simulink model "demo"  (R2021b)
settings: Solver=VariableStepAuto  StartTime=0.0  StopTime=10  RelTol=1e-3
undefined symbols (not defined in the file or in its folder): xc7vx485tffg1157
libraries: hdlBasic x1736, vmcUtilities x1
(part 6 of 7)

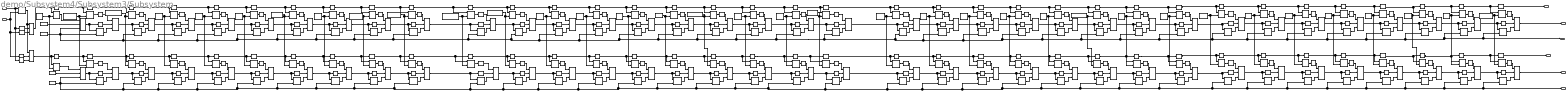
== system demo/Subsystem4/Subsystem3/Subsystem ==
  note: 30
  note: 20
  note: tmp_3
  note: ooki
  note: 10
  note: tmp_2
  note: tiisai
  note: 01
  In1 : Inport
  In2 : Inport  Port=2
  AddSub{,1..17,23..38,41..61,70..79,87,97,108,110..111} (70 alike) : hdlBasic/AddSub  mode=Addition  use_carryin=off  use_carryout=off  en=off  latency=1  precision=User Defined  arith_type="Signed  (2's comp)"  n_bits=32  bin_pt=0  quantization=Truncate  overflow=Wrap  use_behavioral_HDL=off  hw_selection=Fabric  pipelined=off  XmcBlockStatus=1  maskContainerNames=tabcontainer1  block_type=addsub  block_config=sysgen:Addsub_config
  Constant1 : hdlBasic/Constant  const=0  gui_display_data_type=Fixed-point  arith_type=Signed (2's comp)  n_bits=32  bin_pt=0  preci_type=Single  exp_width=8  frac_width=24  explicit_period=on  period=1  XmcBlockStatus=1  maskContainerNames=tabcontainer1  block_type=constant  block_config=sysgen:Constant_config
  Constant2 : hdlBasic/Constant  const=1  gui_display_data_type=Fixed-point  arith_type=Signed (2's comp)  n_bits=32  bin_pt=0  preci_type=Single  exp_width=8  frac_width=24  explicit_period=on  period=1  XmcBlockStatus=1  maskContainerNames=tabcontainer1  block_type=constant  block_config=sysgen:Constant_config
  Constant6 : hdlBasic/Constant  const=0  gui_display_data_type=Fixed-point  arith_type=Signed (2's comp)  n_bits=32  bin_pt=0  preci_type=Single  exp_width=8  frac_width=24  explicit_period=on  period=1  XmcBlockStatus=1  maskContainerNames=tabcontainer1  block_type=constant  block_config=sysgen:Constant_config
  Constant7 : hdlBasic/Constant  const=1  gui_display_data_type=Fixed-point  arith_type=Signed (2's comp)  n_bits=32  bin_pt=0  preci_type=Single  exp_width=8  frac_width=24  explicit_period=on  period=1  XmcBlockStatus=1  maskContainerNames=tabcontainer1  block_type=constant  block_config=sysgen:Constant_config
  Delay{1..7,9..10,12..13,15..16,19..20,22..23,25..26,28..29,31..32,34..35,37..38,41..42,44..45,47..48,50..52,54..56,58,62,64..65,67..68,71..72,74..75,77..78,80..82,84..85,87..88,91..92,94..95,97..98,100..103,105..107,109,114..115,117..118,120..125,127..129,131,133..134,136..138,140..141,143..144,147..148,150..151,153..154,156..158,160..161,163..164,167..168,170..171,173..174,176,188..189,194,205,227,238,257..258,260..261,263..264,266..267,269..270,272..273,275..276,279..280,282..283,285..286,288..290,292,321} (146 alike) : hdlBasic/Delay  rst=off  en=off  latency=1  reg_retiming=off  XmcBlockStatus=1  maskContainerNames=group1  block_type=delay  block_config=sysgen:Delay_config
  Delay{8,11,14,17..18,21,24,27,30,33,36,39..40,43,46,49,53,57,63,66,69..70,73,76,79,83,86,89..90,93,96,99,104,108,116,119,126,130,132,135,139,142,145..146,149,152,155,159,162,165..166,169,172,175,187,216,249,256,259,262,265,268,271,274,277..278,281,284,287,291} (70 alike) : hdlBasic/Delay  rst=off  en=off  latency=2  reg_retiming=off  XmcBlockStatus=1  maskContainerNames=group1  block_type=delay  block_config=sysgen:Delay_config
  Mux{,1..37,40..57,68..77,86,97,106..109} (72 alike) : hdlBasic/Mux  inputs=2  en=off  latency=1  precision=Full  arith_type=Unsigned  n_bits=16  bin_pt=14  quantization=Truncate  overflow=Wrap  XmcBlockStatus=1  maskContainerNames=tabcontainer1  block_type=mux  block_config=sysgen:Mux_config
  Relational : hdlBasic/Relational  mode=a<b  op_type=Bool  en=off  latency=1  XmcBlockStatus=1  maskContainerNames=tabcontainer1  block_type=relational  block_config=sysgen:Relational_config
  Relational{1..36,39..59,70..78,86,97,107..110} (72 alike) : hdlBasic/Relational  mode=a>=b  op_type=Bool  en=off  latency=1  XmcBlockStatus=1  maskContainerNames=tabcontainer1  block_type=relational  block_config=sysgen:Relational_config
  logi_b0 : hdlBasic/Constant  const=-1.0000000000000000000000000000000000000000000000000000000  gui_display_data_type=Floating-point  arith_type=Floating-point  n_bits=8  bin_pt=8  preci_type=Double  exp_width=8  frac_width=24  explicit_period=on  period=1  XmcBlockStatus=1  maskContainerNames=tabcontainer1  block_type=constant  block_config=sysgen:Constant_config
  logi_b1 : hdlBasic/Constant  const=-0.9838709677419354981964261241955682635307312011718750000  gui_display_data_type=Floating-point  arith_type=Floating-point  n_bits=8  bin_pt=8  preci_type=Double  exp_width=8  frac_width=24  explicit_period=on  period=1  XmcBlockStatus=1  maskContainerNames=tabcontainer1  block_type=constant  block_config=sysgen:Constant_config
  logi_b10 : hdlBasic/Constant  const=-0.8387096774193547599196563169243745505809783935546875000  gui_display_data_type=Floating-point  arith_type=Floating-point  n_bits=8  bin_pt=8  preci_type=Double  exp_width=8  frac_width=24  explicit_period=on  period=1  XmcBlockStatus=1  maskContainerNames=tabcontainer1  block_type=constant  block_config=sysgen:Constant_config
  logi_b11 : hdlBasic/Constant  const=-0.8225806451612902581160824411199428141117095947265625000  gui_display_data_type=Floating-point  arith_type=Floating-point  n_bits=8  bin_pt=8  preci_type=Double  exp_width=8  frac_width=24  explicit_period=on  period=1  XmcBlockStatus=1  maskContainerNames=tabcontainer1  block_type=constant  block_config=sysgen:Constant_config
  logi_b12 : hdlBasic/Constant  const=-0.8064516129032257563125085653155110776424407958984375000  gui_display_data_type=Floating-point  arith_type=Floating-point  n_bits=8  bin_pt=8  preci_type=Double  exp_width=8  frac_width=24  explicit_period=on  period=1  XmcBlockStatus=1  maskContainerNames=tabcontainer1  block_type=constant  block_config=sysgen:Constant_config
  logi_b13 : hdlBasic/Constant  const=-0.7903225806451612545089346895110793411731719970703125000  gui_display_data_type=Floating-point  arith_type=Floating-point  n_bits=8  bin_pt=8  preci_type=Double  exp_width=8  frac_width=24  explicit_period=on  period=1  XmcBlockStatus=1  maskContainerNames=tabcontainer1  block_type=constant  block_config=sysgen:Constant_config
  logi_b14 : hdlBasic/Constant  const=-0.7741935483870967527053608137066476047039031982421875000  gui_display_data_type=Floating-point  arith_type=Floating-point  n_bits=8  bin_pt=8  preci_type=Double  exp_width=8  frac_width=24  explicit_period=on  period=1  XmcBlockStatus=1  maskContainerNames=tabcontainer1  block_type=constant  block_config=sysgen:Constant_config
  logi_b15 : hdlBasic/Constant  const=-0.7580645161290322509017869379022158682346343994140625000  gui_display_data_type=Floating-point  arith_type=Floating-point  n_bits=8  bin_pt=8  preci_type=Double  exp_width=8  frac_width=24  explicit_period=on  period=1  XmcBlockStatus=1  maskContainerNames=tabcontainer1  block_type=constant  block_config=sysgen:Constant_config
  logi_b16 : hdlBasic/Constant  const=-0.7419354838709677490982130620977841317653656005859375000  gui_display_data_type=Floating-point  arith_type=Floating-point  n_bits=8  bin_pt=8  preci_type=Double  exp_width=8  frac_width=24  explicit_period=on  period=1  XmcBlockStatus=1  maskContainerNames=tabcontainer1  block_type=constant  block_config=sysgen:Constant_config
  logi_b17 : hdlBasic/Constant  const=-0.7258064516129032472946391862933523952960968017578125000  gui_display_data_type=Floating-point  arith_type=Floating-point  n_bits=8  bin_pt=8  preci_type=Double  exp_width=8  frac_width=24  explicit_period=on  period=1  XmcBlockStatus=1  maskContainerNames=tabcontainer1  block_type=constant  block_config=sysgen:Constant_config
  logi_b18 : hdlBasic/Constant  const=-0.7096774193548387454910653104889206588268280029296875000  gui_display_data_type=Floating-point  arith_type=Floating-point  n_bits=8  bin_pt=8  preci_type=Double  exp_width=8  frac_width=24  explicit_period=on  period=1  XmcBlockStatus=1  maskContainerNames=tabcontainer1  block_type=constant  block_config=sysgen:Constant_config
  logi_b19 : hdlBasic/Constant  const=-0.6935483870967741326651889721688348799943923950195312500  gui_display_data_type=Floating-point  arith_type=Floating-point  n_bits=8  bin_pt=8  preci_type=Double  exp_width=8  frac_width=24  explicit_period=on  period=1  XmcBlockStatus=1  maskContainerNames=tabcontainer1  block_type=constant  block_config=sysgen:Constant_config
  logi_b2 : hdlBasic/Constant  const=-0.9677419354838709963928522483911365270614624023437500000  gui_display_data_type=Floating-point  arith_type=Floating-point  n_bits=8  bin_pt=8  preci_type=Double  exp_width=8  frac_width=24  explicit_period=on  period=1  XmcBlockStatus=1  maskContainerNames=tabcontainer1  block_type=constant  block_config=sysgen:Constant_config
  logi_b20 : hdlBasic/Constant  const=-0.6774193548387096308616150963644031435251235961914062500  gui_display_data_type=Floating-point  arith_type=Floating-point  n_bits=8  bin_pt=8  preci_type=Double  exp_width=8  frac_width=24  explicit_period=on  period=1  XmcBlockStatus=1  maskContainerNames=tabcontainer1  block_type=constant  block_config=sysgen:Constant_config
  logi_b21 : hdlBasic/Constant  const=-0.6612903225806451290580412205599714070558547973632812500  gui_display_data_type=Floating-point  arith_type=Floating-point  n_bits=8  bin_pt=8  preci_type=Double  exp_width=8  frac_width=24  explicit_period=on  period=1  XmcBlockStatus=1  maskContainerNames=tabcontainer1  block_type=constant  block_config=sysgen:Constant_config
  logi_b22 : hdlBasic/Constant  const=-0.6451612903225806272544673447555396705865859985351562500  gui_display_data_type=Floating-point  arith_type=Floating-point  n_bits=8  bin_pt=8  preci_type=Double  exp_width=8  frac_width=24  explicit_period=on  period=1  XmcBlockStatus=1  maskContainerNames=tabcontainer1  block_type=constant  block_config=sysgen:Constant_config
  logi_b23 : hdlBasic/Constant  const=-0.6290322580645161254508934689511079341173171997070312500  gui_display_data_type=Floating-point  arith_type=Floating-point  n_bits=8  bin_pt=8  preci_type=Double  exp_width=8  frac_width=24  explicit_period=on  period=1  XmcBlockStatus=1  maskContainerNames=tabcontainer1  block_type=constant  block_config=sysgen:Constant_config
  logi_b24 : hdlBasic/Constant  const=-0.6129032258064516236473195931466761976480484008789062500  gui_display_data_type=Floating-point  arith_type=Floating-point  n_bits=8  bin_pt=8  preci_type=Double  exp_width=8  frac_width=24  explicit_period=on  period=1  XmcBlockStatus=1  maskContainerNames=tabcontainer1  block_type=constant  block_config=sysgen:Constant_config
  logi_b25 : hdlBasic/Constant  const=-0.5967741935483871218437457173422444611787796020507812500  gui_display_data_type=Floating-point  arith_type=Floating-point  n_bits=8  bin_pt=8  preci_type=Double  exp_width=8  frac_width=24  explicit_period=on  period=1  XmcBlockStatus=1  maskContainerNames=tabcontainer1  block_type=constant  block_config=sysgen:Constant_config
  logi_b26 : hdlBasic/Constant  const=-0.5806451612903225090178693790221586823463439941406250000  gui_display_data_type=Floating-point  arith_type=Floating-point  n_bits=8  bin_pt=8  preci_type=Double  exp_width=8  frac_width=24  explicit_period=on  period=1  XmcBlockStatus=1  maskContainerNames=tabcontainer1  block_type=constant  block_config=sysgen:Constant_config
  logi_b27 : hdlBasic/Constant  const=-0.5645161290322580072142955032177269458770751953125000000  gui_display_data_type=Floating-point  arith_type=Floating-point  n_bits=8  bin_pt=8  preci_type=Double  exp_width=8  frac_width=24  explicit_period=on  period=1  XmcBlockStatus=1  maskContainerNames=tabcontainer1  block_type=constant  block_config=sysgen:Constant_config
  logi_b28 : hdlBasic/Constant  const=-0.5483870967741935054107216274132952094078063964843750000  gui_display_data_type=Floating-point  arith_type=Floating-point  n_bits=8  bin_pt=8  preci_type=Double  exp_width=8  frac_width=24  explicit_period=on  period=1  XmcBlockStatus=1  maskContainerNames=tabcontainer1  block_type=constant  block_config=sysgen:Constant_config
  logi_b29 : hdlBasic/Constant  const=-0.5322580645161290036071477516088634729385375976562500000  gui_display_data_type=Floating-point  arith_type=Floating-point  n_bits=8  bin_pt=8  preci_type=Double  exp_width=8  frac_width=24  explicit_period=on  period=1  XmcBlockStatus=1  maskContainerNames=tabcontainer1  block_type=constant  block_config=sysgen:Constant_config
  logi_b3 : hdlBasic/Constant  const=-0.9516129032258063835669759100710507482290267944335937500  gui_display_data_type=Floating-point  arith_type=Floating-point  n_bits=8  bin_pt=8  preci_type=Double  exp_width=8  frac_width=24  explicit_period=on  period=1  XmcBlockStatus=1  maskContainerNames=tabcontainer1  block_type=constant  block_config=sysgen:Constant_config
  logi_b30 : hdlBasic/Constant  const=-0.5161290322580645018035738758044317364692687988281250000  gui_display_data_type=Floating-point  arith_type=Floating-point  n_bits=8  bin_pt=8  preci_type=Double  exp_width=8  frac_width=24  explicit_period=on  period=1  XmcBlockStatus=1  maskContainerNames=tabcontainer1  block_type=constant  block_config=sysgen:Constant_config
  logi_b31 : hdlBasic/Constant  const=-0.5000000000000000000000000000000000000000000000000000000  gui_display_data_type=Floating-point  arith_type=Floating-point  n_bits=8  bin_pt=8  preci_type=Double  exp_width=8  frac_width=24  explicit_period=on  period=1  XmcBlockStatus=1  maskContainerNames=tabcontainer1  block_type=constant  block_config=sysgen:Constant_config
  logi_b32 : hdlBasic/Constant  const=-0.4838709677419354981964261241955682635307312011718750000  gui_display_data_type=Floating-point  arith_type=Floating-point  n_bits=8  bin_pt=8  preci_type=Double  exp_width=8  frac_width=24  explicit_period=on  period=1  XmcBlockStatus=1  maskContainerNames=tabcontainer1  block_type=constant  block_config=sysgen:Constant_config
  logi_b33 : hdlBasic/Constant  const=-0.4677419354838709408817010171333095058798789978027343750  gui_display_data_type=Floating-point  arith_type=Floating-point  n_bits=8  bin_pt=8  preci_type=Double  exp_width=8  frac_width=24  explicit_period=on  period=1  XmcBlockStatus=1  maskContainerNames=tabcontainer1  block_type=constant  block_config=sysgen:Constant_config
  logi_b34 : hdlBasic/Constant  const=-0.4516129032258064390781271413288777694106101989746093750  gui_display_data_type=Floating-point  arith_type=Floating-point  n_bits=8  bin_pt=8  preci_type=Double  exp_width=8  frac_width=24  explicit_period=on  period=1  XmcBlockStatus=1  maskContainerNames=tabcontainer1  block_type=constant  block_config=sysgen:Constant_config
  logi_b35 : hdlBasic/Constant  const=-0.4354838709677419372745532655244460329413414001464843750  gui_display_data_type=Floating-point  arith_type=Floating-point  n_bits=8  bin_pt=8  preci_type=Double  exp_width=8  frac_width=24  explicit_period=on  period=1  XmcBlockStatus=1  maskContainerNames=tabcontainer1  block_type=constant  block_config=sysgen:Constant_config
  logi_b4 : hdlBasic/Constant  const=-0.9354838709677418817634020342666190117597579956054687500  gui_display_data_type=Floating-point  arith_type=Floating-point  n_bits=8  bin_pt=8  preci_type=Double  exp_width=8  frac_width=24  explicit_period=on  period=1  XmcBlockStatus=1  maskContainerNames=tabcontainer1  block_type=constant  block_config=sysgen:Constant_config
  logi_b5 : hdlBasic/Constant  const=-0.9193548387096773799598281584621872752904891967773437500  gui_display_data_type=Floating-point  arith_type=Floating-point  n_bits=8  bin_pt=8  preci_type=Double  exp_width=8  frac_width=24  explicit_period=on  period=1  XmcBlockStatus=1  maskContainerNames=tabcontainer1  block_type=constant  block_config=sysgen:Constant_config
  logi_b6 : hdlBasic/Constant  const=-0.9032258064516128781562542826577555388212203979492187500  gui_display_data_type=Floating-point  arith_type=Floating-point  n_bits=8  bin_pt=8  preci_type=Double  exp_width=8  frac_width=24  explicit_period=on  period=1  XmcBlockStatus=1  maskContainerNames=tabcontainer1  block_type=constant  block_config=sysgen:Constant_config
  logi_b7 : hdlBasic/Constant  const=-0.8870967741935483763526804068533238023519515991210937500  gui_display_data_type=Floating-point  arith_type=Floating-point  n_bits=8  bin_pt=8  preci_type=Double  exp_width=8  frac_width=24  explicit_period=on  period=1  XmcBlockStatus=1  maskContainerNames=tabcontainer1  block_type=constant  block_config=sysgen:Constant_config
  logi_b8 : hdlBasic/Constant  const=-0.8709677419354838745491065310488920658826828002929687500  gui_display_data_type=Floating-point  arith_type=Floating-point  n_bits=8  bin_pt=8  preci_type=Double  exp_width=8  frac_width=24  explicit_period=on  period=1  XmcBlockStatus=1  maskContainerNames=tabcontainer1  block_type=constant  block_config=sysgen:Constant_config
  logi_b9 : hdlBasic/Constant  const=-0.8548387096774193727455326552444603294134140014648437500  gui_display_data_type=Floating-point  arith_type=Floating-point  n_bits=8  bin_pt=8  preci_type=Double  exp_width=8  frac_width=24  explicit_period=on  period=1  XmcBlockStatus=1  maskContainerNames=tabcontainer1  block_type=constant  block_config=sysgen:Constant_config
  logical_x0 : hdlBasic/Mux  inputs=2  en=off  latency=1  precision=Full  arith_type=Unsigned  n_bits=16  bin_pt=14  quantization=Truncate  overflow=Wrap  XmcBlockStatus=1  maskContainerNames=tabcontainer1  block_type=mux  block_config=sysgen:Mux_config
  logical_y0 : hdlBasic/Mux  inputs=2  en=off  latency=1  precision=Full  arith_type=Unsigned  n_bits=16  bin_pt=14  quantization=Truncate  overflow=Wrap  XmcBlockStatus=1  maskContainerNames=tabcontainer1  block_type=mux  block_config=sysgen:Mux_config
  Out1 : Outport
  Out2 : Outport  Port=2
  Out3 : Outport  Port=3
  Out4 : Outport  Port=4
  Out5 : Outport  Port=5
  Out6 : Outport  Port=6
  wires:
  Delay158/1 -> Mux43/2
  AddSub6/1 -> Mux7/3
  Delay1/1 -> logical_y0/2
  Delay292/1 -> Mux69/1
  Relational2/1 -> Mux/1
  Delay55/1 -> Mux21/1
  Delay100/1 -> Mux31/1
  Delay58/1 -> Mux22/1
  Delay91/1 -> Mux18/1
  Mux52/1 -> AddSub55/1, Delay151/1
  Delay68/1 -> Mux33/2
  Relational5/1 -> Delay15/1
  Delay154/1 -> Mux54/2
  AddSub73/1 -> Mux71/3
  Relational20/1 -> Delay100/1
  Delay124/1 -> Mux42/1
  Relational42/1 -> Delay124/1
  Relational28/1 -> Delay44/1
  Delay117/1 -> Mux41/1
  Delay114/1 -> Mux9/1
  Relational43/1 -> Delay127/1
  Delay141/1 -> Mux50/2
  AddSub15/1 -> Mux17/3
  Delay42/1 -> Mux25/2
  Relational12/1 -> Delay102/1
  AddSub12/1 -> Mux14/3
  Delay104/1 -> Delay83/1, Relational13/1
  Delay56/1 -> Mux21/2
  Relational7/1 -> Delay22/1
  logi_b23/1 -> Relational46/2, Relational53/2
  AddSub24/1 -> Mux22/3
  logi_b21/1 -> Relational44/2, Relational51/2
  Delay105/1 -> Mux15/1
  Delay20/1 -> Mux5/2
  Delay276/1 -> Mux71/2
  Delay92/1 -> Mux18/2
  logi_b15/1 -> Relational17/2, Relational34/2
  Delay153/1 -> Mux54/1
  Relational6/1 -> Delay19/1
  AddSub56/1 -> Mux54/3
  Delay74/1 -> Mux35/1
  Delay37/1 -> Mux24/1
  Delay291/1 -> Out4/1
  AddSub43/1 -> Mux13/3
  Delay5/1 -> Relational1/1, Delay8/1
  Relational50/1 -> Delay122/1
  Mux23/1 -> AddSub26/1, Delay38/1
  Delay137/1 -> Mux56/2
  AddSub9/1 -> Mux11/3
  Mux9/1 -> Delay103/1, AddSub12/1
  Relational58/1 -> Delay133/1
  Delay3/1 -> logical_x0/2
  AddSub25/1 -> Mux23/3
  Delay275/1 -> Mux71/1
  Relational34/1 -> Delay74/1
  AddSub17/1 -> Mux19/3
  Delay160/1 -> Mux44/1
  Mux37/1 -> AddSub42/1, Delay118/1
  Mux33/1 -> AddSub35/1, Delay72/1
  Delay15/1 -> Mux4/1
  Relational45/1 -> Delay163/1
  Mux/1 -> Delay7/1, AddSub/1
  Relational54/1 -> Delay150/1
  Delay263/1 -> Mux107/1
  Delay76/1 -> Relational36/1, Delay79/1
  Delay109/1 -> Mux12/1
  AddSub72/1 -> Mux70/3
  Delay238/1 -> Mux86/2
  AddSub87/1 -> Mux97/3
  AddSub75/1 -> Mux73/3
  Delay64/1 -> Mux32/1
  Relational72/1 -> Delay272/1
  AddSub54/1 -> Mux52/3
  Mux20/1 -> Delay56/1, AddSub23/1
  Delay289/1 -> Mux75/2
  Delay264/1 -> Mux107/2
  Delay205/1 -> Mux77/2
  Delay90/1 -> Delay93/1, Relational17/1
  Relational15/1 -> Delay87/1
  Relational27/1 -> Delay41/1
  Delay34/1 -> Mux23/1
  Delay281/1 -> Delay284/1, Relational76/1
  AddSub52/1 -> Mux51/3
  Mux27/1 -> AddSub30/1, Delay51/1
  AddSub5/1 -> Mux6/3
  Mux30/1 -> AddSub34/1, Delay101/1
  logi_b34/1 -> Relational78/2, Relational110/2
  Delay282/1 -> Mux73/1
  AddSub74/1 -> Mux72/3
  AddSub78/1 -> Mux75/3
  AddSub41/1 -> Mux40/3
  AddSub53/1 -> Mux49/3
  Delay18/1 -> Delay21/1, Relational7/1
  Relational53/1 -> Delay147/1
  In1/1 -> Relational/1, Delay4/1, Delay1/1
  Delay119/1 -> Relational42/1, Delay126/1
  Delay170/1 -> Mux47/1
  Relational77/1 -> Delay321/1
  Delay13/1 -> Mux3/2
  Delay21/1 -> Delay24/1, Relational8/1
  Delay123/1 -> Mux49/2
  Relational78/1 -> Delay288/1
  AddSub10/1 -> Mux12/3
  Delay45/1 -> Mux26/2
  Delay84/1 -> Mux16/1
  Delay227/1 -> Mux86/1
  logi_b13/1 -> Relational15/2, Relational32/2
  Delay48/1 -> Mux27/2
  Delay135/1 -> Delay271/1, Relational71/1
  Delay277/1 -> Delay278/1, Relational74/1
  AddSub42/1 -> Mux41/3
  AddSub50/1 -> Mux47/3
  AddSub30/1 -> Mux28/3
  logi_b30/1 -> Relational73/2, Relational97/2
  Delay174/1 -> Mux48/2
  Relational46/1 -> Delay167/1
  Delay43/1 -> Delay46/1, Relational29/1
  Mux69/1 -> AddSub72/1, Delay273/1
  Delay159/1 -> Relational44/1, Delay162/1
  AddSub46/1 -> Mux43/3
  Mux36/1 -> AddSub38/1, Delay81/1
  logi_b2/1 -> Relational3/2, Relational24/2
  Delay7/1 -> Mux1/2
  Delay134/1 -> Mux57/2
  Delay75/1 -> Mux35/2
  Delay73/1 -> Delay76/1, Relational35/1
  Delay138/1 -> Mux13/2
  Mux51/1 -> AddSub54/1, Delay148/1
  logi_b3/1 -> Relational25/2, Relational4/2
  logi_b32/1 -> Relational75/2, Relational108/2
  Delay125/1 -> Mux42/2
  Mux72/1 -> AddSub75/1, Delay283/1
  AddSub11/1 -> Mux32/3
  Mux74/1 -> AddSub78/1, Delay289/1
  Delay144/1 -> Mux51/2
  Delay187/1 -> Relational86/1, Delay216/1
  Relational8/1 -> Delay25/1
  Mux86/1 -> AddSub87/1, Delay258/1
  AddSub34/1 -> Mux31/3
  Delay17/1 -> Delay18/1, Relational6/1
  Delay27/1 -> Relational22/1, Delay30/1
  Delay166/1 -> Delay169/1, Relational47/1
  Relational14/1 -> Delay84/1
  Delay103/1 -> Mux14/2
  AddSub3/1 -> Mux4/3
  Delay70/1 -> Delay73/1, Relational34/1
  Delay26/1 -> Mux7/2
  Delay268/1 -> Out1/1
  Relational86/1 -> Delay194/1
  logi_b26/1 -> Relational50/2, Relational56/2
  logi_b29/1 -> Relational72/2, Relational86/2
  Delay161/1 -> Mux44/2
  Delay72/1 -> Mux34/2
  Mux29/1 -> Delay107/1, AddSub9/1
  Delay36/1 -> Relational26/1, Delay39/1
  Delay261/1 -> Mux106/2
  logi_b22/1 -> Relational45/2, Relational52/2
  AddSub35/1 -> Mux34/3
  AddSub49/1 -> Mux46/3
  AddSub33/1 -> Mux33/3
  Mux55/1 -> AddSub59/1, Delay134/1
  AddSub70/1 -> Mux77/3
  Mux18/1 -> AddSub17/1, Delay95/1
  Delay269/1 -> Mux76/1
  Delay38/1 -> Mux24/2
  Delay9/1 -> Mux2/1
  Relational11/1 -> Delay106/1
  AddSub2/1 -> Mux3/3
  Delay86/1 -> Relational15/1, Delay89/1
  Delay162/1 -> Relational45/1, Delay165/1
  Delay287/1 -> Relational59/1, Delay291/1
  Delay290/1 -> Mux76/2
  Relational73/1 -> Delay275/1
  Delay81/1 -> Mux37/2
  Delay194/1 -> Mux77/1
  AddSub47/1 -> Mux44/3
  logi_b27/1 -> Relational57/2, Relational58/2
  Delay49/1 -> Relational10/1, Delay53/1
  Delay89/1 -> Delay90/1, Relational16/1
  Relational19/1 -> Delay109/1
  Delay147/1 -> Mux52/1
  logi_b20/1 -> Relational43/2, Relational49/2
  In2/1 -> Relational/2, Delay3/1, Delay2/1
  logical_x0/1 -> Relational23/1, Delay54/1
  Mux1/1 -> AddSub1/1, Delay10/1
  Relational4/1 -> Delay12/1
  Delay78/1 -> Mux36/2
  AddSub45/1 -> Mux42/3
  Delay136/1 -> Mux56/1
  Mux10/1 -> AddSub43/1, Delay138/1
  Delay12/1 -> Mux3/1
  Delay106/1 -> Mux11/1
  Delay57/1 -> Delay33/1, Relational24/1
  Relational18/1 -> Delay97/1
  Relational33/1 -> Delay71/1
  AddSub28/1 -> Mux26/3
  Delay259/1 -> Delay262/1, Relational109/1
  Mux109/1 -> Out5/1
  Relational36/1 -> Delay80/1
  Delay24/1 -> Relational9/1, Delay27/1
  Relational41/1 -> Delay128/1
  Constant7/1 -> AddSub12/2, AddSub45/2, Out6/1, AddSub111/2, AddSub78/2, AddSub76/2, AddSub75/2, AddSub74/2, AddSub73/2, AddSub72/2, AddSub71/2, AddSub58/2, AddSub53/2, AddSub51/2, AddSub50/2, AddSub49/2, AddSub48/2, AddSub47/2, AddSub46/2, AddSub41/2, AddSub34/2, AddSub32/2, AddSub17/2, AddSub16/2, AddSub15/2, AddSub14/2, AddSub13/2, AddSub8/2, AddSub30/2, AddSub29/2, AddSub28/2, AddSub27/2, AddSub26/2, AddSub25/2, AddSub24/2, AddSub23/2, Mux20/3
  Relational/1 -> logical_x0/1, logical_y0/1
  Relational21/1 -> Delay55/1
  logi_b9/1 -> Relational10/2, Relational22/2
  Delay167/1 -> Mux46/1
  AddSub71/1 -> Mux69/3
  Delay127/1 -> Mux43/1
  Delay142/1 -> Relational52/1, Delay145/1
  Mux50/1 -> AddSub52/1, Delay144/1
  Delay168/1 -> Mux46/2
  logi_b33/1 -> Relational76/2, Relational109/2
  Delay122/1 -> Mux49/1
  Relational31/1 -> Delay64/1
  logi_b8/1 -> Relational30/2, Relational9/2
  Delay98/1 -> Mux30/2
  Relational51/1 -> Delay140/1
  Delay116/1 -> Relational41/1, Delay130/1
  Delay53/1 -> Relational12/1, Delay104/1
  Relational17/1 -> Delay94/1
  Relational16/1 -> Delay91/1
  Relational1/1 -> Delay6/1
  Delay65/1 -> Mux32/2
  Constant6/1 -> Mux20/2
  AddSub8/1 -> Mux9/3
  Delay40/1 -> Delay43/1, Relational28/1
  logi_b35/1 -> Relational59/2, Relational70/2
  Delay175/1 -> Relational57/1, Delay135/1
  Mux77/1 -> AddSub77/1, Delay238/1
  Mux56/1 -> Delay270/1, AddSub71/1
  Delay69/1 -> Delay70/1, Relational33/1
  Delay133/1 -> Mux57/1
  Relational10/1 -> Delay114/1
  Mux21/1 -> AddSub24/1, Delay32/1
  Delay163/1 -> Mux45/1
  Relational39/1 -> Delay120/1
  logi_b24/1 -> Relational47/2, Relational54/2
  Delay283/1 -> Mux73/2
  Mux14/1 -> AddSub13/1, Delay82/1
  Mux22/1 -> AddSub25/1, Delay35/1
  Mux49/1 -> AddSub58/1, Delay137/1
  Constant2/1 -> AddSub31/2, AddSub9/2, AddSub11/2, AddSub33/2, AddSub35/2, AddSub36/2, AddSub37/2, AddSub60/2, AddSub44/2, AddSub52/2, AddSub54/2, AddSub55/2, AddSub56/2, AddSub59/2, Out3/1, AddSub79/2, AddSub110/2, AddSub108/2, AddSub97/2, AddSub87/2, AddSub77/2, AddSub70/2, AddSub61/2, AddSub57/2, AddSub43/2, AddSub42/2, AddSub38/2, AddSub10/2, AddSub7/2, AddSub6/2, AddSub5/2, AddSub4/2, AddSub3/2, AddSub2/2, AddSub1/2, AddSub/2, Mux/3
  Delay87/1 -> Mux17/1
  Delay66/1 -> Relational32/1, Delay69/1
  Mux3/1 -> AddSub3/1, Delay16/1
  Delay173/1 -> Mux48/1
  Delay101/1 -> Mux31/2
  Relational44/1 -> Delay160/1
  Delay140/1 -> Mux50/1
  AddSub55/1 -> Mux53/3
  Delay11/1 -> Relational4/1, Delay14/1
  Mux48/1 -> AddSub53/1, Delay123/1
  AddSub77/1 -> Mux86/3
  Relational48/1 -> Delay173/1
  Delay85/1 -> Mux16/2
  Mux57/1 -> Delay176/1, AddSub61/1
  AddSub32/1 -> Mux30/3
  Relational75/1 -> Delay282/1
  logi_b28/1 -> Relational71/2, Relational77/2
  Delay286/1 -> Mux74/2
  Mux26/1 -> AddSub29/1, Delay48/1
  Delay131/1 -> Mux13/1
  Mux43/1 -> AddSub47/1, Delay161/1
  Delay172/1 -> Relational50/1, Delay175/1
  Delay63/1 -> Relational31/1, Delay66/1
  Constant1/1 -> Mux/2
  Mux16/1 -> AddSub15/1, Delay88/1
  logi_b1/1 -> Relational21/2, Relational1/2
  Delay23/1 -> Mux6/2
  Mux106/1 -> AddSub108/1, Delay264/1
  Mux47/1 -> AddSub51/1, Delay174/1
  Delay156/1 -> Mux55/1
  Delay288/1 -> Mux75/1
  Mux76/1 -> Out2/1
  Mux53/1 -> AddSub56/1, Delay154/1
  Delay4/1 -> logical_x0/3
  Delay164/1 -> Mux45/2
  Relational26/1 -> Delay37/1
  Relational32/1 -> Delay67/1
  Delay29/1 -> Mux8/2
  Delay31/1 -> Mux29/1
  Delay169/1 -> Delay172/1, Relational48/1
  Relational22/1 -> Delay31/1
  Delay155/1 -> Relational58/1, Delay132/1
  logi_b25/1 -> Relational48/2, Relational55/2
  Delay52/1 -> Mux29/2
  Delay50/1 -> Mux28/1
  Relational47/1 -> Delay170/1
  Delay266/1 -> Mux108/1
  Delay278/1 -> Delay281/1, Relational75/1
  Relational59/1 -> Delay188/1
  Delay271/1 -> Relational72/1, Delay274/1
  Mux44/1 -> AddSub48/1, Delay164/1
  logi_b31/1 -> Relational74/2, Relational107/2
  Relational3/1 -> Delay9/1
  Delay189/1 -> Mux109/2
  Relational40/1 -> Delay117/1
  Delay257/1 -> Mux97/1
  Mux108/1 -> AddSub79/1, Delay290/1
  Delay79/1 -> Relational40/1, Delay116/1
  logi_b10/1 -> Relational12/2, Relational11/2
  Mux107/1 -> AddSub110/1, Delay267/1
  logical_y0/1 -> Relational2/1, Delay5/1
  Delay35/1 -> Mux23/2
  AddSub13/1 -> Mux15/3
  AddSub31/1 -> Mux29/3
  Delay71/1 -> Mux34/1
  Delay83/1 -> Relational14/1, Delay86/1
  AddSub37/1 -> Mux36/3
  Delay284/1 -> Relational78/1, Delay287/1
  Delay33/1 -> Relational25/1, Delay36/1
  AddSub/1 -> Mux1/3
  Delay262/1 -> Relational110/1, Delay265/1
  Mux35/1 -> AddSub37/1, Delay78/1
  Delay97/1 -> Mux30/1
  Mux17/1 -> AddSub16/1, Delay92/1
  Relational29/1 -> Delay47/1
  Delay94/1 -> Mux19/1
  Delay130/1 -> Delay139/1, Relational49/1
  logi_b16/1 -> Relational18/2, Relational35/2
  Delay165/1 -> Delay166/1, Relational46/1
  Mux75/1 -> AddSub111/1, Delay189/1
  Delay150/1 -> Mux53/1
  Mux8/1 -> AddSub31/1, Delay52/1
  Mux24/1 -> AddSub27/1, Delay42/1
  AddSub14/1 -> Mux16/3
  Mux32/1 -> AddSub33/1, Delay68/1
  logi_b19/1 -> Relational42/2, Relational41/2
  logi_b12/1 -> Relational14/2, Relational31/2
  AddSub97/1 -> Mux106/3
  Relational70/1 -> Delay269/1
  AddSub110/1 -> Mux108/3
  Delay39/1 -> Delay40/1, Relational27/1
  Relational107/1 -> Delay257/1
  Delay149/1 -> Delay152/1, Relational55/1
  Mux42/1 -> AddSub46/1, Delay158/1
  Mux34/1 -> AddSub36/1, Delay75/1
  Relational23/1 -> Mux20/1
  Delay67/1 -> Mux33/1
  Delay32/1 -> Mux22/2
  AddSub79/1 -> Mux76/3
  Mux31/1 -> AddSub41/1, Delay121/1
  Delay62/1 -> Mux12/2
  Mux2/1 -> AddSub2/1, Delay13/1
  Delay120/1 -> Mux40/1
  AddSub61/1 -> Mux68/3
  Delay6/1 -> Mux1/1
  Mux97/1 -> AddSub97/1, Delay261/1
  Mux5/1 -> AddSub5/1, Delay23/1
  Delay279/1 -> Mux72/1
  Relational30/1 -> Delay50/1
  Delay128/1 -> Mux10/1
  Mux45/1 -> AddSub49/1, Delay168/1
  Relational74/1 -> Delay279/1
  AddSub1/1 -> Mux2/3
  Delay129/1 -> Mux10/2
  Mux11/1 -> AddSub10/1, Delay62/1
  Delay132/1 -> Delay187/1, Relational77/1
  Delay258/1 -> Mux97/2
  AddSub51/1 -> Mux48/3
  Delay2/1 -> logical_y0/3
  logi_b6/1 -> Relational28/2, Relational7/2
  Mux28/1 -> AddSub8/1, Delay115/1
  AddSub26/1 -> Mux24/3
  Mux25/1 -> AddSub28/1, Delay45/1
  Delay41/1 -> Mux25/1
  Delay118/1 -> Mux41/2
  Relational49/1 -> Delay131/1
  AddSub4/1 -> Mux5/3
  Delay146/1 -> Delay149/1, Relational54/1
  Delay25/1 -> Mux7/1
  Delay176/1 -> Mux68/2
  Delay19/1 -> Mux5/1
  Delay285/1 -> Mux74/1
  Delay171/1 -> Mux47/2
  Delay148/1 -> Mux52/2
  Delay99/1 -> Relational39/1, Delay119/1
  Delay216/1 -> Relational97/1, Delay249/1
  Delay107/1 -> Mux11/2
  Delay108/1 -> Delay63/1, Relational19/1
  Mux71/1 -> AddSub74/1, Delay280/1
  Delay188/1 -> Mux109/1
  logi_b14/1 -> Relational16/2, Relational33/2
  Mux54/1 -> AddSub57/1, Delay157/1
  Mux15/1 -> AddSub14/1, Delay85/1
  Delay321/1 -> Mux68/1
  AddSub108/1 -> Mux107/3
  Delay44/1 -> Mux26/1
  AddSub48/1 -> Mux45/3
  Delay273/1 -> Mux70/2
  Mux12/1 -> AddSub11/1, Delay65/1
  Relational55/1 -> Delay153/1
  Delay47/1 -> Mux27/1
  Delay51/1 -> Mux28/2
  Mux13/1 -> AddSub44/1, Delay141/1
  AddSub23/1 -> Mux21/3
  Mux7/1 -> AddSub7/1, Delay29/1
  Delay143/1 -> Mux51/1
  Delay96/1 -> Relational20/1, Delay99/1
  Delay256/1 -> Delay259/1, Relational108/1
  Delay272/1 -> Mux70/1
  Relational97/1 -> Delay227/1
  Delay8/1 -> Relational3/1, Delay11/1
  Relational109/1 -> Delay263/1
  Mux70/1 -> AddSub73/1, Delay276/1
  Relational57/1 -> Delay136/1
  Delay280/1 -> Mux72/2
  Relational76/1 -> Delay285/1
  Delay126/1 -> Delay159/1, Relational43/1
  logi_b11/1 -> Relational13/2, Relational19/2
  Delay82/1 -> Mux15/2
  Delay95/1 -> Mux19/2
  Delay54/1 -> Delay57/1, Relational21/1
  Relational56/1 -> Delay156/1
  Mux41/1 -> Delay129/1, AddSub60/1
  Delay265/1 -> Relational70/1, Delay268/1
  Delay270/1 -> Mux69/2
  logi_b17/1 -> Relational20/2, Relational36/2
  Relational108/1 -> Delay260/1
  AddSub59/1 -> Mux57/3
  Delay93/1 -> Delay96/1, Relational18/1
  Delay22/1 -> Mux6/1
  AddSub111/1 -> Mux109/3
  AddSub36/1 -> Mux35/3
  Mux68/1 -> AddSub70/1, Delay205/1
  AddSub57/1 -> Mux55/3
  Relational71/1 -> Delay292/1
  Delay46/1 -> Relational30/1, Delay49/1
  AddSub58/1 -> Mux56/3
  AddSub7/1 -> Mux8/3
  Mux19/1 -> AddSub32/1, Delay98/1
  Delay152/1 -> Relational56/1, Delay155/1
  Delay14/1 -> Relational5/1, Delay17/1
  Delay88/1 -> Mux17/2
  Delay16/1 -> Mux4/2
  Delay10/1 -> Mux2/2
  Delay267/1 -> Mux108/2
  Relational110/1 -> Delay266/1
  Delay121/1 -> Mux40/2
  Mux73/1 -> AddSub76/1, Delay286/1
  Relational35/1 -> Delay77/1
  Delay30/1 -> Relational11/1, Delay108/1
  Mux4/1 -> AddSub4/1, Delay20/1
  Delay260/1 -> Mux106/1
  AddSub38/1 -> Mux37/3
  Delay274/1 -> Relational73/1, Delay277/1
  Delay102/1 -> Mux14/1
  AddSub16/1 -> Mux18/3
  Delay139/1 -> Relational51/1, Delay142/1
  Mux46/1 -> AddSub50/1, Delay171/1
  AddSub27/1 -> Mux25/3
  logi_b5/1 -> Relational27/2, Relational6/2
  Relational25/1 -> Delay34/1
  Relational52/1 -> Delay143/1
  Delay115/1 -> Mux9/2
  Delay157/1 -> Mux55/2
  Delay145/1 -> Delay146/1, Relational53/1
  Mux6/1 -> AddSub6/1, Delay26/1
  logi_b0/1 -> Relational23/2, Relational2/2
  logi_b7/1 -> Relational29/2, Relational8/2
  AddSub60/1 -> Mux10/3
  Delay80/1 -> Mux37/1
  Delay77/1 -> Mux36/1
  Delay28/1 -> Mux8/1
  Relational9/1 -> Delay28/1
  AddSub76/1 -> Mux74/3
  Mux40/1 -> Delay125/1, AddSub45/1
  Relational24/1 -> Delay58/1
  Delay249/1 -> Delay256/1, Relational107/1
  Delay151/1 -> Mux53/2
  AddSub44/1 -> Mux50/3
  logi_b18/1 -> Relational39/2, Relational40/2
  logi_b4/1 -> Relational26/2, Relational5/2
  Relational13/1 -> Delay105/1
  AddSub29/1 -> Mux27/3
